simulink model "CruiseControl"  (R2021a)
settings: Solver=VariableStepAuto  StartTime=0.0  StopTime=40  RelTol=1e-3
libraries: simulink x9, pid_lib x2
settings Model: Creator=david  LastModifiedBy=david
settings SolverCC: ZeroCrossAlgorithm=Adaptive
settings DebuggingCC: IgnoredZcDiagnostic=none

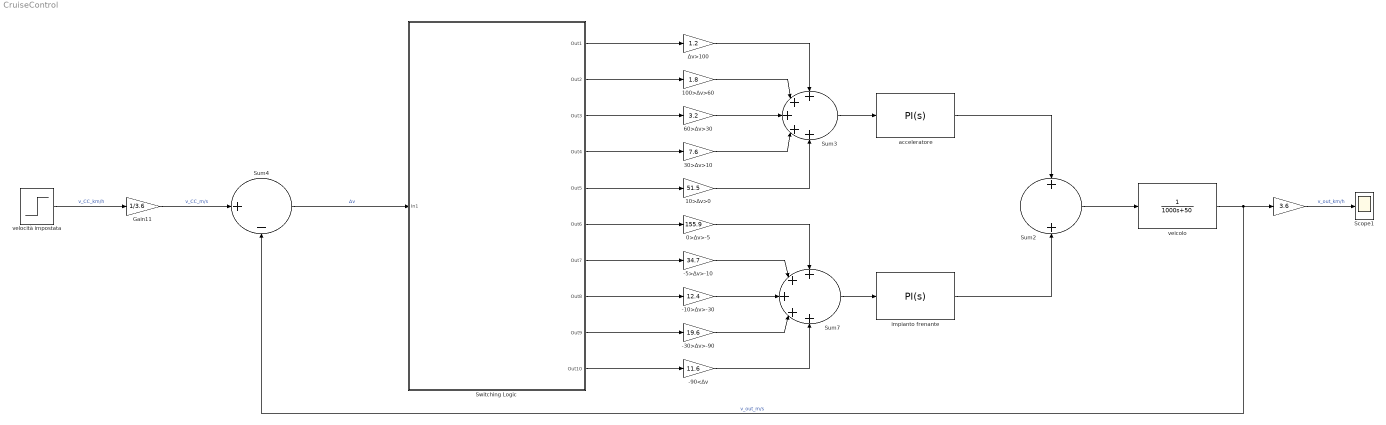
== system CruiseControl ==
  " " : Gain  Gain=3.6
  -10>Δv>-30 : Gain  Gain=12.4
  -30>Δv>-90 : Gain  Gain=19.6
  -5>Δv>-10 : Gain  Gain=34.7
  -90<Δv : Gain  Gain=11.6
  0>Δv>-5 : Gain  Gain=155.9
  100>Δv>60 : Gain  Gain=1.8
  10>Δv>0 : Gain  Gain=51.5
  30>Δv>10 : Gain  Gain=7.6
  60>Δv>30 : Gain  Gain=3.2
  Gain11 : Gain  Gain=1/3.6
  Scope1 : Scope
  Sum2 : Sum
  Sum3 : Sum  Inputs=+++++
  Sum4 : Sum  Inputs=|+-
  Sum7 : Sum  Inputs=+++++
  Switching Logic : Subsystem
  acceleratore : pid_lib/PID Controller  Controller=PI  Form=Parallel  TimeDomain=Continuous-time  UseExternalTs=off  SampleTime=-1  IntegratorMethod=Forward Euler  FilterMethod=Forward Euler  ControllerParametersSource=internal  P=20  I=1  D=0  UseFilter=on  N=100  TunerSelectOption=Transfer Function Based (PID Tuner App)  InitialConditionSource=internal  InitialConditionForIntegrator=0  InitialConditionForFilter=0  DifferentiatorICPrevScaledInput=0  ExternalReset=none  TrackingMode=off  Kt=1  LimitOutput=off  SatLimitsSource=internal  UpperSaturationLimit=inf  LowerSaturationLimit=-inf  LinearizeAsGain=on  AntiWindupMode=none  Kb=1  POutMin=[]  POutMax=[]  IOutMin=[]  IOutMax=[]  DOutMin=[]  DOutMax=[]  NOutMin=[]  NOutMax=[]  SumOutMin=[]  SumOutMax=[]  SaturationOutMin=[]  SaturationOutMax=[]  PParamMin=[]  PParamMax=[]  IParamMin=[]  IParamMax=[]  DParamMin=[]  DParamMax=[]  NParamMin=[]  NParamMax=[]  KbParamMin=[]  KbParamMax=[]  KtParamMin=[]  KtParamMax=[]  KbOutMin=[]  KbOutMax=[]  KtOutMin=[]  KtOutMax=[]  IntegratorOutMin=[]  IntegratorOutMax=[]  FilterOutMin=[]  FilterOutMax=[]  SumI1OutMin=[]  SumI1OutMax=[]  SumI2OutMin=[]  SumI2OutMax=[]  SumI3OutMin=[]  SumI3OutMax=[]  SumI4OutMin=[]  SumI4OutMax=[]  SumDOutMin=[]  SumDOutMax=[]  DifferentiatorOutMin=[]  DifferentiatorOutMax=[]  FilterDiffOutCoefMin=[]  FilterDiffOutCoefMax=[]  ReciprocalOutMin=[]  ReciprocalOutMax=[]  SumDenOutMin=[]  SumDenOutMax=[]  SumNumOutMin=[]  SumNumOutMax=[]  DivideOutMin=[]  DivideOutMax=[]  UdiffTsProdOutMin=[]  UdiffTsProdOutMax=[]  NTsProdOutMin=[]  NTsProdOutMax=[]  UintegralTsProdOutMin=[]  UintegralTsProdOutMax=[]  UngainTsProdOutMin=[]  UngainTsProdOutMax=[]  IntegratorContinuousStateAttributes=''  IntegratorStateMustResolveToSignalObject=off  IntegratorRTWStateStorageClass=Auto  FilterContinuousStateAttributes=''  FilterStateMustResolveToSignalObject=off  FilterRTWStateStorageClass=Auto  ParallelPVariant=InternalParameters  IdealPVariant=Disabled  IVariant=InternalParameters  DVariant=Disabled  IntegratorVariant=Continuous  SatVariant=Disabled  AWVariant=Passthrough  PCopyVariant=Disabled  TRVariant=Disabled  FdbkBlocksVariant=Forward  IdealPFdbkVariant=Disabled  SatFdbkVariant=Disabled  DerivativeFilterVariant=Disabled  NVariant=Disabled  NCopyVariant=Disabled_SignalSpec  FilterICVariant=Disabled  IntegratorICVariant=InternalICs  ExternalResetVariant=Disabled  TRSumVariant=Passthrough  SumFdbkVariant=Disabled  SumVariant=Sum_PI  TsampFilterVariant=InternalTs  TsampNgainVariant=Passthrough  TsampIntegralVariant=Passthrough  ExternalSaturationOutDataTypeStr=Inherit: Same as second input
  impianto frenante : pid_lib/PID Controller  Controller=PI  Form=Parallel  TimeDomain=Continuous-time  UseExternalTs=off  SampleTime=-1  IntegratorMethod=Forward Euler  FilterMethod=Forward Euler  ControllerParametersSource=internal  P=20  I=1  D=0  UseFilter=on  N=100  TunerSelectOption=Transfer Function Based (PID Tuner App)  InitialConditionSource=internal  InitialConditionForIntegrator=0  InitialConditionForFilter=0  DifferentiatorICPrevScaledInput=0  ExternalReset=none  TrackingMode=off  Kt=1  LimitOutput=off  SatLimitsSource=internal  UpperSaturationLimit=inf  LowerSaturationLimit=-inf  LinearizeAsGain=on  AntiWindupMode=none  Kb=1  POutMin=[]  POutMax=[]  IOutMin=[]  IOutMax=[]  DOutMin=[]  DOutMax=[]  NOutMin=[]  NOutMax=[]  SumOutMin=[]  SumOutMax=[]  SaturationOutMin=[]  SaturationOutMax=[]  PParamMin=[]  PParamMax=[]  IParamMin=[]  IParamMax=[]  DParamMin=[]  DParamMax=[]  NParamMin=[]  NParamMax=[]  KbParamMin=[]  KbParamMax=[]  KtParamMin=[]  KtParamMax=[]  KbOutMin=[]  KbOutMax=[]  KtOutMin=[]  KtOutMax=[]  IntegratorOutMin=[]  IntegratorOutMax=[]  FilterOutMin=[]  FilterOutMax=[]  SumI1OutMin=[]  SumI1OutMax=[]  SumI2OutMin=[]  SumI2OutMax=[]  SumI3OutMin=[]  SumI3OutMax=[]  SumI4OutMin=[]  SumI4OutMax=[]  SumDOutMin=[]  SumDOutMax=[]  DifferentiatorOutMin=[]  DifferentiatorOutMax=[]  FilterDiffOutCoefMin=[]  FilterDiffOutCoefMax=[]  ReciprocalOutMin=[]  ReciprocalOutMax=[]  SumDenOutMin=[]  SumDenOutMax=[]  SumNumOutMin=[]  SumNumOutMax=[]  DivideOutMin=[]  DivideOutMax=[]  UdiffTsProdOutMin=[]  UdiffTsProdOutMax=[]  NTsProdOutMin=[]  NTsProdOutMax=[]  UintegralTsProdOutMin=[]  UintegralTsProdOutMax=[]  UngainTsProdOutMin=[]  UngainTsProdOutMax=[]  IntegratorContinuousStateAttributes=''  IntegratorStateMustResolveToSignalObject=off  IntegratorRTWStateStorageClass=Auto  FilterContinuousStateAttributes=''  FilterStateMustResolveToSignalObject=off  FilterRTWStateStorageClass=Auto  ParallelPVariant=InternalParameters  IdealPVariant=Disabled  IVariant=InternalParameters  DVariant=Disabled  IntegratorVariant=Continuous  SatVariant=Disabled  AWVariant=Passthrough  PCopyVariant=Disabled  TRVariant=Disabled  FdbkBlocksVariant=Forward  IdealPFdbkVariant=Disabled  SatFdbkVariant=Disabled  DerivativeFilterVariant=Disabled  NVariant=Disabled  NCopyVariant=Disabled_SignalSpec  FilterICVariant=Disabled  IntegratorICVariant=InternalICs  ExternalResetVariant=Disabled  TRSumVariant=Passthrough  SumFdbkVariant=Disabled  SumVariant=Sum_PI  TsampFilterVariant=InternalTs  TsampNgainVariant=Passthrough  TsampIntegralVariant=Passthrough  ExternalSaturationOutDataTypeStr=Inherit: Same as second input
  veicolo : TransferFcn  Denominator=[1000 50]
  velocità impostata : Step  After=110  SampleTime=0.1
  Δv>100 : Gain  Gain=1.2
  wires:
  " "/1 -> Scope1/1  "v_out_km/h"
  veicolo/1 -> Sum4/2, " "/1  "v_out_m/s"
  Gain11/1 -> Sum4/1  "v_CC_m/s"
  velocità impostata/1 -> Gain11/1  "v_CC_km/h"
  Switching Logic/2(Out2) -> 100>Δv>60/1
  Switching Logic/4(Out4) -> 30>Δv>10/1
  Switching Logic/1(Out1) -> Δv>100/1
  Switching Logic/3(Out3) -> 60>Δv>30/1
  acceleratore/1 -> Sum2/1
  10>Δv>0/1 -> Sum3/5
  60>Δv>30/1 -> Sum3/3
  Δv>100/1 -> Sum3/1
  30>Δv>10/1 -> Sum3/4
  Switching Logic/5(Out5) -> 10>Δv>0/1
  Sum3/1 -> acceleratore/1
  Sum4/1 -> Switching Logic/1(In1)  "Δv"
  100>Δv>60/1 -> Sum3/2
  Switching Logic/7(Out7) -> -5>Δv>-10/1
  -90<Δv/1 -> Sum7/5
  Switching Logic/6(Out6) -> 0>Δv>-5/1
  Sum7/1 -> impianto frenante/1
  Switching Logic/9(Out9) -> -30>Δv>-90/1
  -30>Δv>-90/1 -> Sum7/4
  Switching Logic/8(Out8) -> -10>Δv>-30/1
  impianto frenante/1 -> Sum2/2
  Switching Logic/10(Out10) -> -90<Δv/1
  0>Δv>-5/1 -> Sum7/1
  -10>Δv>-30/1 -> Sum7/3
  -5>Δv>-10/1 -> Sum7/2
  Sum2/1 -> veicolo/1

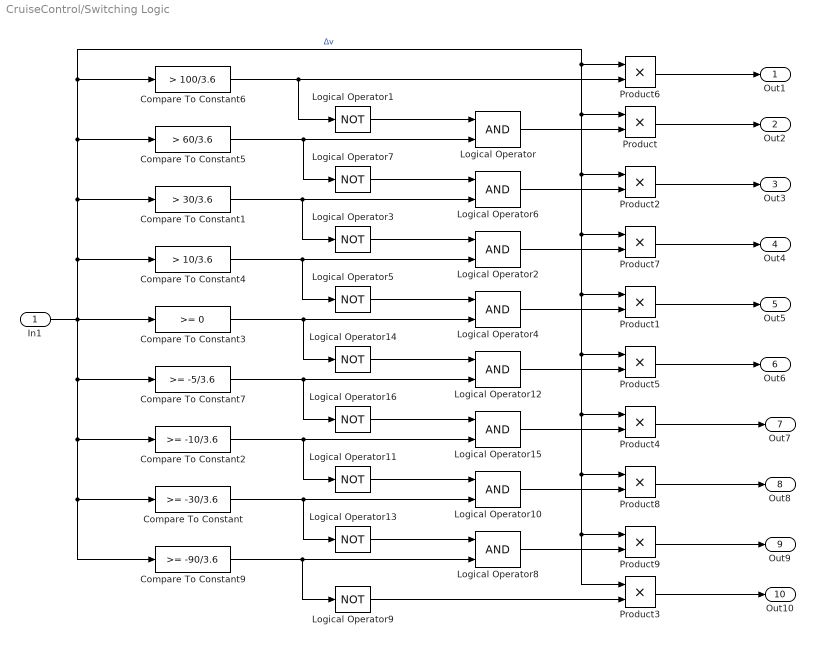
== system CruiseControl/Switching Logic ==
  In1 : Inport
  Compare To Constant : simulink/Logic and Bit Operations/Compare To Constant  relop=>=  const=-30/3.6  OutDataTypeStr=boolean
  Compare To Constant1 : simulink/Logic and Bit Operations/Compare To Constant  relop=>  const=30/3.6  OutDataTypeStr=boolean
  Compare To Constant2 : simulink/Logic and Bit Operations/Compare To Constant  relop=>=  const=-10/3.6  OutDataTypeStr=boolean
  Compare To Constant3 : simulink/Logic and Bit Operations/Compare To Constant  relop=>=  const=0  OutDataTypeStr=boolean
  Compare To Constant4 : simulink/Logic and Bit Operations/Compare To Constant  relop=>  const=10/3.6  OutDataTypeStr=boolean
  Compare To Constant5 : simulink/Logic and Bit Operations/Compare To Constant  relop=>  const=60/3.6  OutDataTypeStr=boolean
  Compare To Constant6 : simulink/Logic and Bit Operations/Compare To Constant  relop=>  const=100/3.6  OutDataTypeStr=boolean
  Compare To Constant7 : simulink/Logic and Bit Operations/Compare To Constant  relop=>=  const=-5/3.6  OutDataTypeStr=boolean
  Compare To Constant9 : simulink/Logic and Bit Operations/Compare To Constant  relop=>=  const=-90/3.6  OutDataTypeStr=boolean
  Logical Operator{,2,4,6,8,10,12,15} (8 alike) : Logic  AllPortsSameDT=off  OutDataTypeStr=boolean
  Logical Operator{1,3,5,7,9,11,13..14,16} (9 alike) : Logic  Operator=NOT  AllPortsSameDT=off  OutDataTypeStr=boolean
  Product{,1..9} (10 alike) : Product
  Out1 : Outport
  Out2 : Outport  Port=2
  Out3 : Outport  Port=3
  Out4 : Outport  Port=4
  Out5 : Outport  Port=5
  Out6 : Outport  Port=6
  Out7 : Outport  Port=7
  Out8 : Outport  Port=8
  Out9 : Outport  Port=9
  Out10 : Outport  Port=10
  wires:
  Compare To Constant1/1 -> Logical Operator3/1, Logical Operator6/2
  Logical Operator6/1 -> Product2/2
  Compare To Constant3/1 -> Logical Operator14/1, Logical Operator4/2
  Logical Operator1/1 -> Logical Operator/1
  Product2/1 -> Out3/1
  Product6/1 -> Out1/1
  Logical Operator/1 -> Product/2
  Compare To Constant5/1 -> Logical Operator7/1, Logical Operator/2
  Product1/1 -> Out5/1
  Logical Operator7/1 -> Logical Operator6/1
  Logical Operator2/1 -> Product7/2
  Compare To Constant4/1 -> Logical Operator5/1, Logical Operator2/2
  Logical Operator4/1 -> Product1/2
  Logical Operator3/1 -> Logical Operator2/1
  Logical Operator5/1 -> Logical Operator4/1
  Compare To Constant6/1 -> Product6/2, Logical Operator1/1
  Product/1 -> Out2/1
  Product7/1 -> Out4/1
  Logical Operator9/1 -> Product3/2
  Logical Operator10/1 -> Product8/2
  Product5/1 -> Out6/1
  Product4/1 -> Out7/1
  Logical Operator13/1 -> Logical Operator8/1
  Compare To Constant9/1 -> Logical Operator9/1, Logical Operator8/2
  Logical Operator15/1 -> Product4/2
  Product3/1 -> Out10/1
  Logical Operator16/1 -> Logical Operator15/1
  Product9/1 -> Out9/1
  Logical Operator8/1 -> Product9/2
  In1/1 -> Compare To Constant5/1, Compare To Constant6/1, Product/1, Product2/1, Product7/1, Product3/1, Product9/1, Product8/1, Product4/1, Product5/1, Product1/1, Product6/1, Compare To Constant1/1, Compare To Constant4/1, Compare To Constant9/1, Compare To Constant/1, Compare To Constant2/1, Compare To Constant7/1, Compare To Constant3/1  "Δv"
  Logical Operator12/1 -> Product5/2
  Compare To Constant/1 -> Logical Operator13/1, Logical Operator10/2
  Logical Operator14/1 -> Logical Operator12/1
  Logical Operator11/1 -> Logical Operator10/1
  Compare To Constant7/1 -> Logical Operator16/1, Logical Operator12/2
  Compare To Constant2/1 -> Logical Operator11/1, Logical Operator15/2
  Product8/1 -> Out8/1
